simulink model "debug_version"  (Simulink 7.6)
settings: Solver=FixedStepDiscrete  StartTime=0.0  StopTime=inf  FixedStep=0.05  RelTol=1e-3
StartFcn:
  | tic
undefined symbols (not defined in the file or in its folder): DiscIntNeverNeededParam
libraries: realtime_pacer_lib x2, simulink x2, qbmove_library x2
settings Model: Creator=Michele  LastModifiedBy=Administrator

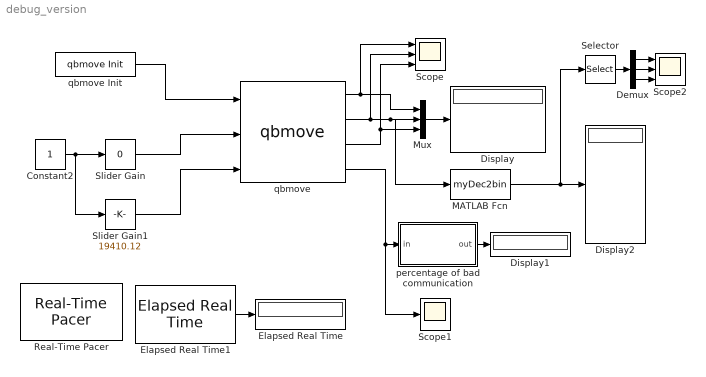
== system debug_version ==
  Constant2 : Constant
  Demux : Demux  Outputs=3
  Display : Display
  Display1 : Display
  Display2 : Display
  Elapsed Real Time : Display
      settings: Decimation=2
  Elapsed Real Time1 : realtime_pacer_lib/Elapsed Real Time
  MATLAB Fcn : MATLABFcn  MATLABFcn=myDec2bin
  Mux : Mux  Inputs=3
  Real-Time Pacer : realtime_pacer_lib/Real-Time Pacer  simTimePerRealTime=1
  Scope : Scope  NumInputPorts=3
      settings: YMin=0~38~-1  YMax=4500~38~1
  Scope1 : Scope
      settings: YMin=-1  YMax=1
  Scope2 : Scope  NumInputPorts=3
      settings: YMin=1~-1~-1  YMax=1~1~1  SaveName=ScopeData2
  Selector : Selector  IndexOptions=Index vector (dialog)  Indices=[1 2 3]  OutputSizes=1
  Slider Gain : simulink/Math Operations/Slider Gain  SystemSampleTime=-1  low=-30000  gain=0  high=30000
  Slider Gain1 : simulink/Math Operations/Slider Gain  SystemSampleTime=-1  low=-30000  gain=19410.12  high=30000
  percentage of bad communication : Subsystem
  qbmove : qbmove_library/qbmove  ID=65  ACTIVE_COMM_DIRECTIONS=Both  PSoC_MODE=Equilibrium Position and Stiffness Preset  DAISY_CHAINING=off  MAX_ANG=30000  SW_LIMIT=inf  OFFSET=0
  qbmove Init : qbmove_library/qbmove Init  NUMBER_OF_COM=1
  wires:
  Constant2/1 -> Slider Gain/1, Slider Gain1/1
  qbmove Init/1 -> qbmove/1
  Slider Gain/1 -> qbmove/2
  Slider Gain1/1 -> qbmove/3
  Elapsed Real Time1/1 -> Elapsed Real Time/1
  Mux/1 -> Display/1
  qbmove/1 -> Mux/1, Scope/1
  qbmove/2 -> Scope/2, Mux/2, MATLAB Fcn/1
  qbmove/3 -> Mux/3, Scope/3
  qbmove/4 -> Scope1/1, percentage of bad communication/1(in)
  percentage of bad communication/1(out) -> Display1/1
  MATLAB Fcn/1 -> Display2/1, Selector/1
  Selector/1 -> Demux/1
  Demux/1 -> Scope2/1
  Demux/2 -> Scope2/2
  Demux/3 -> Scope2/3

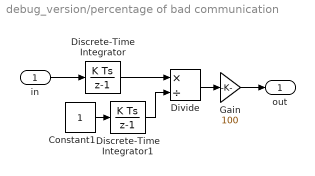
== system debug_version/percentage of bad communication ==
  in : Inport
  Constant1 : Constant
  Discrete-Time Integrator : DiscreteIntegrator  SampleTime=-1  ICPrevOutput=DiscIntNeverNeededParam  ICPrevScaledInput=DiscIntNeverNeededParam
  Discrete-Time Integrator1 : DiscreteIntegrator  SampleTime=-1  ICPrevOutput=DiscIntNeverNeededParam  ICPrevScaledInput=DiscIntNeverNeededParam
  Divide : Product  Inputs=*/
  Gain : Gain  Gain=100
  out : Outport
  wires:
  Divide/1 -> Gain/1
  Discrete-Time Integrator/1 -> Divide/1
  Constant1/1 -> Discrete-Time Integrator1/1
  Discrete-Time Integrator1/1 -> Divide/2
  in/1 -> Discrete-Time Integrator/1
  Gain/1 -> out/1
